simulink model "lab_2_demo"  (R2021a)
settings: Solver=VariableStepAuto  StartTime=0.0  StopTime=50  MaxStep=1e-3  RelTol=1e-3
libraries: pid_lib x1
settings Model: Creator=Artun  LastModifiedBy=Artun

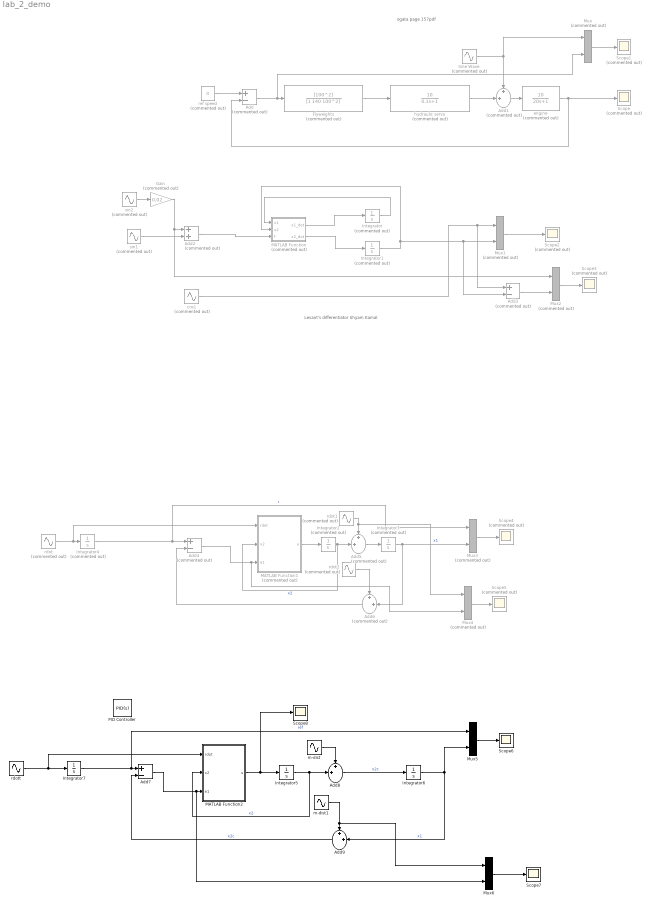
== system lab_2_demo ==
  note: ogata page 157pdf
  note: Levant's differentiator Shyam Kamal
  Add : Sum  Commented=on  Inputs=+-
  Add1 : Sum  Commented=on  Inputs=++|
  Add2 : Sum  Commented=on
  Add3 : Sum  Commented=on  Inputs=+-
  Add4 : Sum  Commented=on  Inputs=+-
  Add5 : Sum  Commented=on  Inputs=++|
  Add6 : Sum  Commented=on  Inputs=++|
  Add7 : Sum  Inputs=+-
  Add8 : Sum  Inputs=++|
  Add9 : Sum  Inputs=++|
  Flyweights : TransferFcn  Commented=on  Numerator=[100^2]  Denominator=[1 140 100^2]
  Gain : Gain  Commented=on  Gain=0.02
  Integrator{,1..4} (5 alike) : Integrator  Commented=on
  Integrator5 : Integrator
  Integrator6 : Integrator
  Integrator7 : Integrator
  MATLAB Function : MATLAB Function  Commented=on  TreatAsAtomicUnit=on
  MATLAB Function1 : MATLAB Function  Commented=on  TreatAsAtomicUnit=on
  MATLAB Function2 : MATLAB Function  TreatAsAtomicUnit=on
  Mux{,1..4} (5 alike) : Mux  Commented=on  Inputs=2
  Mux5 : Mux  Inputs=2
  Mux6 : Mux  Inputs=2
  PID Controller : pid_lib/PID Controller  Controller=PID  Form=Parallel  TimeDomain=Continuous-time  UseExternalTs=off  SampleTime=-1  IntegratorMethod=Forward Euler  FilterMethod=Forward Euler  ControllerParametersSource=internal  P=1  I=1  D=0  UseFilter=on  N=100  TunerSelectOption=Transfer Function Based (PID Tuner App)  InitialConditionSource=internal  InitialConditionForIntegrator=0  InitialConditionForFilter=0  DifferentiatorICPrevScaledInput=0  ExternalReset=none  TrackingMode=off  Kt=1  LimitOutput=off  SatLimitsSource=internal  UpperSaturationLimit=inf  LowerSaturationLimit=-inf  LinearizeAsGain=on  AntiWindupMode=none  Kb=1  POutMin=[]  POutMax=[]  IOutMin=[]  IOutMax=[]  DOutMin=[]  DOutMax=[]  NOutMin=[]  NOutMax=[]  SumOutMin=[]  SumOutMax=[]  SaturationOutMin=[]  SaturationOutMax=[]  PParamMin=[]  PParamMax=[]  IParamMin=[]  IParamMax=[]  DParamMin=[]  DParamMax=[]  NParamMin=[]  NParamMax=[]  KbParamMin=[]  KbParamMax=[]  KtParamMin=[]  KtParamMax=[]  KbOutMin=[]  KbOutMax=[]  KtOutMin=[]  KtOutMax=[]  IntegratorOutMin=[]  IntegratorOutMax=[]  FilterOutMin=[]  FilterOutMax=[]  SumI1OutMin=[]  SumI1OutMax=[]  SumI2OutMin=[]  SumI2OutMax=[]  SumI3OutMin=[]  SumI3OutMax=[]  SumI4OutMin=[]  SumI4OutMax=[]  SumDOutMin=[]  SumDOutMax=[]  DifferentiatorOutMin=[]  DifferentiatorOutMax=[]  FilterDiffOutCoefMin=[]  FilterDiffOutCoefMax=[]  ReciprocalOutMin=[]  ReciprocalOutMax=[]  SumDenOutMin=[]  SumDenOutMax=[]  SumNumOutMin=[]  SumNumOutMax=[]  DivideOutMin=[]  DivideOutMax=[]  UdiffTsProdOutMin=[]  UdiffTsProdOutMax=[]  NTsProdOutMin=[]  NTsProdOutMax=[]  UintegralTsProdOutMin=[]  UintegralTsProdOutMax=[]  UngainTsProdOutMin=[]  UngainTsProdOutMax=[]  IntegratorContinuousStateAttributes=''  IntegratorStateMustResolveToSignalObject=off  IntegratorRTWStateStorageClass=Auto  FilterContinuousStateAttributes=''  FilterStateMustResolveToSignalObject=off  FilterRTWStateStorageClass=Auto  ParallelPVariant=InternalParameters  IdealPVariant=Disabled  IVariant=InternalParameters  DVariant=InternalParameters  IntegratorVariant=Continuous  SatVariant=Disabled  AWVariant=Passthrough  PCopyVariant=Disabled  TRVariant=Disabled  FdbkBlocksVariant=Forward  IdealPFdbkVariant=Disabled  SatFdbkVariant=Disabled  DerivativeFilterVariant=ContFilter  NVariant=InternalParameters  NCopyVariant=Disabled  FilterICVariant=InternalICsFilter  IntegratorICVariant=InternalICs  ExternalResetVariant=Disabled  TRSumVariant=Passthrough  SumFdbkVariant=Disabled  SumVariant=Sum_PID  TsampFilterVariant=InternalTs  TsampNgainVariant=Passthrough  TsampIntegralVariant=Passthrough  ExternalSaturationOutDataTypeStr=Inherit: Same as second input
  Scope{,1..5} (6 alike) : Scope  Commented=on
  Scope6 : Scope
  Scope7 : Scope
  Scope8 : Scope
  Sine Wave : Sin  Commented=on  Amplitude=0.1  Frequency=2*pi*1  SampleTime=0
  cos1 : Sin  Commented=on  Phase=pi/2  SampleTime=0
  engine : TransferFcn  Commented=on  Numerator=[10]  Denominator=[20 1]
  hydraulic servo : TransferFcn  Commented=on  Numerator=[10]  Denominator=[0.1 1]
  m-dist : Sin  Amplitude=5  Frequency=2*pi*(10)  Phase=pi/2  SampleTime=0
  m-dist1 : Sin  Amplitude=0.1  Frequency=2*pi*(10)  Phase=pi/2  SampleTime=0
  rdot : Sin  Commented=on  Frequency=2*pi*(0.1)  Phase=pi/2  SampleTime=0
  rdot1 : Sin  Commented=on  Amplitude=10  Frequency=2*pi*(10)  Phase=pi/2  SampleTime=0
  rdot2 : Sin  Commented=on  Amplitude=0.001  Frequency=2*pi*(15)  Phase=pi/2  SampleTime=0
  rdott : Sin  Frequency=2*pi*(0.1)  Phase=pi/2  SampleTime=0
  ref speed : Constant  Commented=on  Value=0
  sin1 : Sin  Commented=on  SampleTime=0
  sin2 : Sin  Commented=on  Frequency=100  SampleTime=0
  wires:
  ref speed/1 -> Add/1
  hydraulic servo/1 -> Add1/2
  Sine Wave/1 -> Mux/1, Add1/1
  Add/1 -> Mux/2, Flyweights/1
  Flyweights/1 -> hydraulic servo/1
  Add1/1 -> engine/1
  engine/1 -> Add/2, Scope/1
  Mux/1 -> Scope1/1
  MATLAB Function/1(x1_dot) -> Integrator/1
  MATLAB Function/2(x2_dot) -> Integrator1/1
  Integrator/1 -> MATLAB Function/1(x1)
  Integrator1/1 -> Add3/2, Mux1/2, MATLAB Function/2(x2)
  sin1/1 -> Add2/2
  Mux1/1 -> Scope2/1
  cos1/1 -> Add3/1, Mux1/1
  sin2/1 -> Gain/1
  Add2/1 -> MATLAB Function/3(f)
  Add3/1 -> Mux2/2
  Mux2/1 -> Scope3/1
  Gain/1 -> Mux2/1, Add2/1
  Integrator2/1 -> Add5/2, MATLAB Function1/2(x2)  "x2"
  MATLAB Function1/1(u) -> Integrator2/1
  Mux3/1 -> Scope4/1
  Integrator3/1 -> Add6/2, Mux3/2  "x1"
  Add4/1 -> Mux4/2, MATLAB Function1/3(e1)
  rdot/1 -> MATLAB Function1/1(rdot), Integrator4/1
  Integrator4/1 -> Mux3/1, Add4/1  "r"
  Add5/1 -> Integrator3/1
  rdot1/1 -> Mux4/1, Add5/1
  rdot2/1 -> Add6/1
  Add6/1 -> Add4/2
  Mux4/1 -> Scope5/1
  Add8/1 -> Integrator6/1  "x2c"
  Integrator7/1 -> Mux5/1, Add7/1  "ref"
  rdott/1 -> MATLAB Function2/1(rdot), Integrator7/1
  Integrator6/1 -> Add9/2, Mux5/2  "x1"
  Add7/1 -> Mux6/2, MATLAB Function2/3(e1)
  MATLAB Function2/1(u) -> Scope8/1, Integrator5/1
  Mux5/1 -> Scope6/1
  Integrator5/1 -> MATLAB Function2/2(x2), Add8/2  "x2"
  m-dist/1 -> Add8/1
  Mux6/1 -> Scope7/1
  m-dist1/1 -> Mux6/1, Add9/1
  Add9/1 -> Add7/2  "x2c"

== matlab function lab_2_demo/MATLAB Function1 ==
  data: rdot input; u output; x2 input; e1 input
function u  = fcn(rdot,x2,e1)
k=0.5;

u=(rdot-x2)+k*sign(e1+[(rdot-x2)]);

== matlab function lab_2_demo/MATLAB Function ==
  data: x1 input; x1_dot output; x2 input; f input; x2_dot output
function [x1_dot,x2_dot] = fcn(x1,x2,f)
delta0=1.1;
k1=1.5*sqrt(delta0);
k2=1.1*sqrt(delta0);

x1_dot=-k1*sqrt(abs(x1-f))*sign(x1-f)+x2;
x2_dot=-k2*sign(x1-f);

== matlab function lab_2_demo/MATLAB Function2 ==
  data: rdot input; u output; x2 input; e1 input
function u  = fcn(rdot,x2,e1)
k=0.5;

u=(rdot-x2)+k*sign(e1+[(rdot-x2)]);
